simulink model "CMOS_Kernel_Memory_Sync"  (R2023b)
settings: Solver=VariableStepAuto  StartTime=0.0  StopTime=30000000  RelTol=1e-3
values from neighbouring files (symbols this model uses):
  AmountOfPixelsPerScanline = 400    [Kernel_Setup_Script.m]
  AmountOfRamBlocksScanlines = 5    [Kernel_Setup_Script.m]
  AmountOfRamBlocksScanlinesOffset = AmountOfRamBlocksScanlines - 1    (= 4)    [Kernel_Setup_Script.m]
  AmountOfScanlinePixels = 73700    [Kernel_Setup_Script.m]
  AmountOfScanlinePixelsOffset = AmountOfScanlinePixels - 1    (= 73699)    [Kernel_Setup_Script.m]
  AmountOfScanlines = 1100    [Kernel_Setup_Script.m]
  AmountOfScanlinesOffset = AmountOfScanlines - 1    (= 1099)    [Kernel_Setup_Script.m]
  AOPPK_Off = AmountOfPixelsPerScanline - 1    (= 399)    [Kernel_Setup_Script.m]
  AOPPS_Off = AmountOfPixelsPerScanline - 1    (= 399)    [Kernel_Setup_Script.m]
  FramePackOff_0 = FramePackOff_0 - ScanlineFifoCheck    [Kernel_Setup_Script.m]
  FramePackOff_1 = FramePackOff_1 - ScanlineFifoCheck    [Kernel_Setup_Script.m]
  FramePackOff_2 = FramePackOff_2 - ScanlineFifoCheck    [Kernel_Setup_Script.m]
  FramePackOff_3 = FramePackOff_3 - ScanlineFifoCheck    [Kernel_Setup_Script.m]
  FramePackOff_4 = FramePackOff_4 - ScanlineFifoCheck    [Kernel_Setup_Script.m]
  FramePackOff_5 = FramePackOff_5 - ScanlineFifoCheck    [Kernel_Setup_Script.m]
  KernelPackOff_0 = KernelPackOff_0 - KernelBitsPerRow    [Kernel_Setup_Script.m]
  KernelPackOff_1 = KernelPackOff_1 - KernelBitsPerRow    [Kernel_Setup_Script.m]
  KernelPackOff_2 = KernelPackOff_2 - KernelBitsPerRow    [Kernel_Setup_Script.m]
  KernelPackOff_3 = KernelPackOff_3 - KernelBitsPerRow    [Kernel_Setup_Script.m]
  Slice59DownTo48Top = (MsbOffset - (ScanlinePixelBitSizeController*1))    (= 59)    [Kernel_Setup_Script.m]
  Slice71DownTo60Top = (MsbOffset - (ScanlinePixelBitSizeController*0))    (= 71)    [Kernel_Setup_Script.m]
  TotalSectionsForFrames = AmountOfScanlines/AmountOfRamBlocksScanlines    (= 220)    [Kernel_Setup_Script.m]
  UltraRamRows = AmountOfPixelsPerScanline/ScanlineFifoCheck    [Kernel_Setup_Script.m]
  UltraRamRowsCeil = ceil(AmountOfPixelsPerScanline/ScanlineFifoCheck)    [Kernel_Setup_Script.m]
  UltraRamRowsKernel = AmountOfPixelsPerScanline/KernelBitsPerRow    (= 100)    [Kernel_Setup_Script.m]
  UltraRamRowsKernelCeil = ceil(AmountOfPixelsPerScanline/KernelBitsPerRow)    [Kernel_Setup_Script.m]
  UltraRamRowsMemorySectionOffset = UltraRamRowsCeil*AmountOfRamBlocksScanlines    [Kernel_Setup_Script.m]
  UltraRamRowsOffset = UltraRamRowsCeil - 1    [Kernel_Setup_Script.m]
undefined symbols (not defined in the file or in its folder): c, Down, sfvc784, Up, xck26
libraries: hdlBasic x4512, vmcUtilities x1
(part 12 of 39)

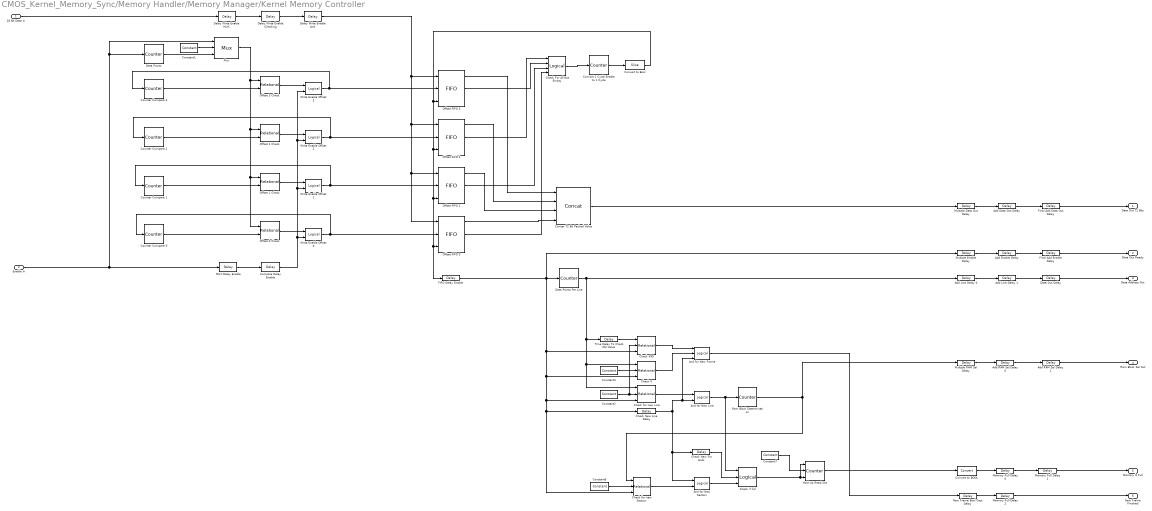
== system CMOS_Kernel_Memory_Sync/Memory Handler/Memory Manager/Kernel Memory Controller ==
  18 Bit Data In : Inport
  Enable In : Inport  Port=2
  Add Data Out Delay : hdlBasic/Delay  rst=off  en=off  latency=1  reg_retiming=off  XmcBlockStatus=1  maskContainerNames=group1  block_type=delay  block_config=sysgen:Delay_config
  Add Enable Delay : hdlBasic/Delay  rst=off  en=off  latency=1  reg_retiming=off  XmcBlockStatus=1  maskContainerNames=group1  block_type=delay  block_config=sysgen:Delay_config
  Add Line Delay 0 : hdlBasic/Delay  rst=off  en=off  latency=3  reg_retiming=off  XmcBlockStatus=1  maskContainerNames=group1  block_type=delay  block_config=sysgen:Delay_config
  Add Line Delay 1 : hdlBasic/Delay  rst=off  en=off  latency=1  reg_retiming=off  XmcBlockStatus=1  maskContainerNames=group1  block_type=delay  block_config=sysgen:Delay_config
  Add RAM Sel Delay 0 : hdlBasic/Delay  rst=off  en=off  latency=1  reg_retiming=off  XmcBlockStatus=1  maskContainerNames=group1  block_type=delay  block_config=sysgen:Delay_config
  Add RAM Sel Delay 1 : hdlBasic/Delay  rst=off  en=off  latency=1  reg_retiming=off  XmcBlockStatus=1  maskContainerNames=group1  block_type=delay  block_config=sysgen:Delay_config
  And for New Frame : hdlBasic/Logical  logical_function=AND  inputs=3  en=off  latency=1  precision=Full  arith_type=Unsigned  n_bits=16  bin_pt=0  align_bp=on  overflow=[]  quantization=[]  XmcBlockStatus=1  maskContainerNames=tabcontainer1  block_type=logical  block_config=sysgen:Logical_config
  And for New Line : hdlBasic/Logical  logical_function=AND  inputs=2  en=off  latency=1  precision=Full  arith_type=Unsigned  n_bits=16  bin_pt=0  align_bp=on  overflow=[]  quantization=[]  XmcBlockStatus=1  maskContainerNames=tabcontainer1  block_type=logical  block_config=sysgen:Logical_config
  And for New Section : hdlBasic/Logical  logical_function=AND  inputs=2  en=off  latency=1  precision=Full  arith_type=Unsigned  n_bits=16  bin_pt=0  align_bp=on  overflow=[]  quantization=[]  XmcBlockStatus=1  maskContainerNames=tabcontainer1  block_type=logical  block_config=sysgen:Logical_config
  Check 0 : hdlBasic/Relational  mode=a=b  op_type=Bool  en=on  latency=1  XmcBlockStatus=1  maskContainerNames=tabcontainer1  block_type=relational  block_config=sysgen:Relational_config
  Check 499 : hdlBasic/Relational  mode=a=b  op_type=Bool  en=on  latency=1  XmcBlockStatus=1  maskContainerNames=tabcontainer1  block_type=relational  block_config=sysgen:Relational_config
  Check For All Not Empty : hdlBasic/Logical  logical_function=NOR  inputs=4  en=off  latency=1  precision=Full  arith_type=Unsigned  n_bits=16  bin_pt=0  align_bp=on  overflow=[]  quantization=[]  XmcBlockStatus=1  maskContainerNames=tabcontainer1  block_type=logical  block_config=sysgen:Logical_config
  Check New For Ands : hdlBasic/Delay  rst=off  en=off  latency=1  reg_retiming=off  XmcBlockStatus=1  maskContainerNames=group1  block_type=delay  block_config=sysgen:Delay_config
  Check New Line Delay : hdlBasic/Delay  rst=off  en=off  latency=1  reg_retiming=off  XmcBlockStatus=1  maskContainerNames=group1  block_type=delay  block_config=sysgen:Delay_config
  Check for new Line : hdlBasic/Relational  mode=a=b  op_type=Bool  en=on  latency=1  XmcBlockStatus=1  maskContainerNames=tabcontainer1  block_type=relational  block_config=sysgen:Relational_config
  Check for new Section : hdlBasic/Relational  mode=a=b  op_type=Bool  en=on  latency=1  XmcBlockStatus=1  maskContainerNames=tabcontainer1  block_type=relational  block_config=sysgen:Relational_config
  Check if full : hdlBasic/Logical  logical_function=AND  inputs=3  en=off  latency=1  precision=Full  arith_type=Unsigned  n_bits=16  bin_pt=0  align_bp=on  overflow=[]  quantization=[]  XmcBlockStatus=1  maskContainerNames=tabcontainer1  block_type=logical  block_config=sysgen:Logical_config
  Compare Delay Enable : hdlBasic/Delay  rst=off  en=off  latency=1  reg_retiming=off  XmcBlockStatus=1  maskContainerNames=group1  block_type=delay  block_config=sysgen:Delay_config
  Concat 72 Bit Packed Value : hdlBasic/Concat  num_inputs=4  XmcBlockStatus=1  maskContainerNames=group1  block_type=concat  block_config=sysgen:Concat_config
  Constant1 : hdlBasic/Constant  const=AOPPK_Off + 1  gui_display_data_type=Fixed-point  arith_type=Unsigned  n_bits=ceil(log2(AmountOfPixelsPerScanline + 1))  bin_pt=0  preci_type=Single  exp_width=8  frac_width=24  explicit_period=off  period=1  XmcBlockStatus=1  maskContainerNames=tabcontainer1  block_type=constant  block_config=sysgen:Constant_config
  Constant2 : hdlBasic/Constant  const=499  gui_display_data_type=Fixed-point  arith_type=Unsigned  n_bits=ceil(log2(UltraRamRowsKernel))+5  bin_pt=0  preci_type=Single  exp_width=8  frac_width=24  explicit_period=off  period=1  XmcBlockStatus=1  maskContainerNames=tabcontainer1  block_type=constant  block_config=sysgen:Constant_config
  Constant3 : hdlBasic/Constant  const=0  gui_display_data_type=Fixed-point  arith_type=Unsigned  n_bits=1  bin_pt=0  preci_type=Single  exp_width=8  frac_width=24  explicit_period=off  period=1  XmcBlockStatus=1  maskContainerNames=tabcontainer1  block_type=constant  block_config=sysgen:Constant_config
  Constant6 : hdlBasic/Constant  const=AmountOfRamBlocksScanlinesOffset  gui_display_data_type=Fixed-point  arith_type=Unsigned  n_bits=ceil(log2(AmountOfRamBlocksScanlines))  bin_pt=0  preci_type=Single  exp_width=8  frac_width=24  explicit_period=off  period=1  XmcBlockStatus=1  maskContainerNames=tabcontainer1  block_type=constant  block_config=sysgen:Constant_config
  Constant7 : hdlBasic/Constant  const=1  gui_display_data_type=Fixed-point  arith_type=Unsigned  n_bits=1  bin_pt=0  preci_type=Single  exp_width=8  frac_width=24  explicit_period=off  period=1  XmcBlockStatus=1  maskContainerNames=tabcontainer1  block_type=constant  block_config=sysgen:Constant_config
  Convert 2 Cycle Enable to 1 Cycle : hdlBasic/Counter  cnt_type=Count limited  cnt_to=2  operation=Up  start_count=0  cnt_by_val=1  arith_type=Unsigned  n_bits=2  bin_pt=0  load_pin=off  rst=off  en=on  explicit_period=Explicit  period=1  use_behavioral_HDL=off  implementation=Fabric  XmcBlockStatus=1  maskContainerNames=group1  block_type=counter  block_config=sysgen:Counter_config  block_width=531  block_height=1023
  Convert to BOOL : hdlBasic/Convert  gui_display_data_type=Boolean  arith_type=Boolean  n_bits=16  bin_pt=14  float_type=Single  exp_bits=8  fraction_bits=24  quantization=Truncate  overflow=Wrap  en=off  latency=3  pipeline=off  XmcBlockStatus=1  maskContainerNames=group2  block_type=convert  block_config=sysgen:Convert_config  block_width=595  block_height=885
  Convert to Bool : hdlBasic/Slice  nbits=1  boolean_output=on  mode=Upper Bit Location + Width  bit1=0  base1=LSB of Input  bit0=0  base0=LSB of Input  XmcBlockStatus=1  maskContainerNames=group1  block_type=slice  block_config=sysgen:Slice_config
  "Counter Compare 0  " : hdlBasic/Counter  cnt_type=Count limited  cnt_to=KernelPackOff_0  operation=Up  start_count=0  cnt_by_val=4  arith_type=Unsigned  n_bits=ceil(log2(KernelPackOff_0+1))  bin_pt=0  load_pin=off  rst=off  en=on  explicit_period=Explicit  period=1  use_behavioral_HDL=off  implementation=Fabric  XmcBlockStatus=1  maskContainerNames=group1  block_type=counter  block_config=sysgen:Counter_config  block_width=531  block_height=1023
  Counter Compare 1 : hdlBasic/Counter  cnt_type=Count limited  cnt_to=KernelPackOff_1  operation=Up  start_count=1  cnt_by_val=4  arith_type=Unsigned  n_bits=ceil(log2(KernelPackOff_1+1))  bin_pt=0  load_pin=off  rst=off  en=on  explicit_period=Explicit  period=1  use_behavioral_HDL=off  implementation=Fabric  XmcBlockStatus=1  maskContainerNames=group1  block_type=counter  block_config=sysgen:Counter_config  block_width=531  block_height=1023
  Counter Compare 2 : hdlBasic/Counter  cnt_type=Count limited  cnt_to=KernelPackOff_2  operation=Up  start_count=2  cnt_by_val=4  arith_type=Unsigned  n_bits=ceil(log2(KernelPackOff_2+1))  bin_pt=0  load_pin=off  rst=off  en=on  explicit_period=Explicit  period=1  use_behavioral_HDL=off  implementation=Fabric  XmcBlockStatus=1  maskContainerNames=group1  block_type=counter  block_config=sysgen:Counter_config  block_width=531  block_height=1023
  Counter Compare 3 : hdlBasic/Counter  cnt_type=Count limited  cnt_to=KernelPackOff_3  operation=Up  start_count=3  cnt_by_val=4  arith_type=Unsigned  n_bits=ceil(log2(KernelPackOff_3+1))  bin_pt=0  load_pin=off  rst=off  en=on  explicit_period=Explicit  period=1  use_behavioral_HDL=off  implementation=Fabric  XmcBlockStatus=1  maskContainerNames=group1  block_type=counter  block_config=sysgen:Counter_config  block_width=531  block_height=1023
  Data Out Delay : hdlBasic/Delay  rst=off  en=off  latency=1  reg_retiming=off  XmcBlockStatus=1  maskContainerNames=group1  block_type=delay  block_config=sysgen:Delay_config
  Data Points : hdlBasic/Counter  cnt_type=Count limited  cnt_to=AOPPK_Off  operation=Up  start_count=0  cnt_by_val=1  arith_type=Unsigned  n_bits=ceil(log2(AmountOfPixelsPerScanline))  bin_pt=0  load_pin=off  rst=off  en=on  explicit_period=Explicit  period=1  use_behavioral_HDL=off  implementation=Fabric  XmcBlockStatus=1  maskContainerNames=group1  block_type=counter  block_config=sysgen:Counter_config  block_width=531  block_height=1023
  Data Points Per Line : hdlBasic/Counter  cnt_type=Count limited  cnt_to=499  operation=Up  start_count=0  cnt_by_val=1  arith_type=Unsigned  n_bits=ceil(log2(UltraRamRowsKernel)) +2  bin_pt=0  load_pin=off  rst=off  en=on  explicit_period=Explicit  period=1  use_behavioral_HDL=off  implementation=Fabric  XmcBlockStatus=1  maskContainerNames=group1  block_type=counter  block_config=sysgen:Counter_config  block_width=531  block_height=1023
  Delay Write Enable And : hdlBasic/Delay  rst=off  en=off  latency=1  reg_retiming=off  XmcBlockStatus=1  maskContainerNames=group1  block_type=delay  block_config=sysgen:Delay_config
  Delay Write Enable Checking : hdlBasic/Delay  rst=off  en=off  latency=1  reg_retiming=off  XmcBlockStatus=1  maskContainerNames=group1  block_type=delay  block_config=sysgen:Delay_config
  Delay Write Enable MUX : hdlBasic/Delay  rst=off  en=off  latency=1  reg_retiming=off  XmcBlockStatus=1  maskContainerNames=group1  block_type=delay  block_config=sysgen:Delay_config
  FIFO Delay Enable : hdlBasic/Delay  rst=off  en=off  latency=1  reg_retiming=off  XmcBlockStatus=1  maskContainerNames=group1  block_type=delay  block_config=sysgen:Delay_config
  Final Add Data Out Delay : hdlBasic/Delay  rst=off  en=off  latency=1  reg_retiming=off  XmcBlockStatus=1  maskContainerNames=group1  block_type=delay  block_config=sysgen:Delay_config
  Final Add Enable Delay : hdlBasic/Delay  rst=off  en=off  latency=1  reg_retiming=off  XmcBlockStatus=1  maskContainerNames=group1  block_type=delay  block_config=sysgen:Delay_config
  Hold Up Read Out : hdlBasic/Counter  cnt_type=Free running  cnt_to=1  operation=Up  start_count=0  cnt_by_val=1  arith_type=Unsigned  n_bits=1  bin_pt=0  load_pin=on  rst=off  en=on  explicit_period=Explicit  period=1  use_behavioral_HDL=off  implementation=Fabric  XmcBlockStatus=1  maskContainerNames=group1  block_type=counter  block_config=sysgen:Counter_config  block_width=531  block_height=1023
  MUX Delay Enable : hdlBasic/Delay  rst=off  en=off  latency=1  reg_retiming=off  XmcBlockStatus=1  maskContainerNames=group1  block_type=delay  block_config=sysgen:Delay_config
  Memory Full Delay 0 : hdlBasic/Delay  rst=off  en=off  latency=1  reg_retiming=off  XmcBlockStatus=1  maskContainerNames=group1  block_type=delay  block_config=sysgen:Delay_config
  Memory Full Delay 1 : hdlBasic/Delay  rst=off  en=off  latency=1  reg_retiming=off  XmcBlockStatus=1  maskContainerNames=group1  block_type=delay  block_config=sysgen:Delay_config
  Memory Full Delay 2 : hdlBasic/Delay  rst=off  en=off  latency=1  reg_retiming=off  XmcBlockStatus=1  maskContainerNames=group1  block_type=delay  block_config=sysgen:Delay_config
  Multiple Data Out Delay : hdlBasic/Delay  rst=off  en=off  latency=3  reg_retiming=off  XmcBlockStatus=1  maskContainerNames=group1  block_type=delay  block_config=sysgen:Delay_config
  Multiple Enable Delay : hdlBasic/Delay  rst=off  en=off  latency=3  reg_retiming=off  XmcBlockStatus=1  maskContainerNames=group1  block_type=delay  block_config=sysgen:Delay_config
  Multiple RAM Sel Delay : hdlBasic/Delay  rst=off  en=off  latency=3  reg_retiming=off  XmcBlockStatus=1  maskContainerNames=group1  block_type=delay  block_config=sysgen:Delay_config
  Mux : hdlBasic/Mux  inputs=2  en=off  latency=1  precision=Full  arith_type=Unsigned  n_bits=16  bin_pt=14  quantization=Truncate  overflow=Wrap  XmcBlockStatus=1  maskContainerNames=tabcontainer1  block_type=mux  block_config=sysgen:Mux_config
  New Frame Bool Cast Delay : hdlBasic/Delay  rst=off  en=off  latency=3  reg_retiming=off  XmcBlockStatus=1  maskContainerNames=group1  block_type=delay  block_config=sysgen:Delay_config
  Offset 0 Check : hdlBasic/Relational  mode=a=b  op_type=Bool  en=off  latency=1  XmcBlockStatus=1  maskContainerNames=tabcontainer1  block_type=relational  block_config=sysgen:Relational_config
  Offset 1 Check : hdlBasic/Relational  mode=a=b  op_type=Bool  en=off  latency=1  XmcBlockStatus=1  maskContainerNames=tabcontainer1  block_type=relational  block_config=sysgen:Relational_config
  Offset 2 Check : hdlBasic/Relational  mode=a=b  op_type=Bool  en=off  latency=1  XmcBlockStatus=1  maskContainerNames=tabcontainer1  block_type=relational  block_config=sysgen:Relational_config
  Offset 3 Check : hdlBasic/Relational  mode=a=b  op_type=Bool  en=off  latency=1  XmcBlockStatus=1  maskContainerNames=tabcontainer1  block_type=relational  block_config=sysgen:Relational_config
  Offset FIFO {0..3} (4 alike) : hdlBasic/FIFO  mem_type=Block RAM  performance_options=Standard_FIFO  embedded_registers=off  depth=16  use_asym_data_widths=off  asym_read_width=32  percent_nbits=4  rst=off  rst_latency=2  en=off  use_dcount=off  use_percent_full_port=off  use_almost_empty=off  almost_empty_thresh=2  use_almost_full=off  use_rd_rst_busy=off  use_wr_rst_busy=off  almost_full_thresh=14  almost_empty_offset=[]  almost_full_offset=[]  explicit_period=off  period=[]  store_only_valid=[]  init_zero=[]  simulation_type=fast_sim  XmcBlockStatus=1  maskContainerNames=tabcontainer1  block_type=fifo  block_config=sysgen:FIFO_config  block_width=538  block_height=997
      settings: infoedit=[]
  Ram Block Determination : hdlBasic/Counter  cnt_type=Count limited  cnt_to=AmountOfRamBlocksScanlinesOffset  operation=Up  start_count=0  cnt_by_val=1  arith_type=Unsigned  n_bits=ceil(log2(AmountOfRamBlocksScanlines))  bin_pt=0  load_pin=off  rst=off  en=on  explicit_period=Explicit  period=1  use_behavioral_HDL=off  implementation=Fabric  XmcBlockStatus=1  maskContainerNames=group1  block_type=counter  block_config=sysgen:Counter_config  block_width=531  block_height=1023
  Time Delay To Check Old Value : hdlBasic/Delay  rst=off  en=off  latency=3  reg_retiming=off  XmcBlockStatus=1  maskContainerNames=group1  block_type=delay  block_config=sysgen:Delay_config
  Write Enable Offset {0..3} (4 alike) : hdlBasic/Logical  logical_function=AND  inputs=2  en=off  latency=1  precision=Full  arith_type=Unsigned  n_bits=16  bin_pt=0  align_bp=on  overflow=[]  quantization=[]  XmcBlockStatus=1  maskContainerNames=tabcontainer1  block_type=logical  block_config=sysgen:Logical_config
  Data Out 72 Bits : Outport
  Data Out Ready : Outport  Port=2
  Data Address Out : Outport  Port=3
  Ram Block Sel Out : Outport  Port=4
  Memory Is Full : Outport  Port=5
  New Frame Finished : Outport  Port=6
  wires:
  FIFO Delay Enable/1 -> Multiple Enable Delay/1, Check 499/3, Check 0/3, Check for new Line/3, Check New Line Delay/1, Check for new Section/3, Data Points Per Line/1
  Add RAM Sel Delay 1/1 -> Ram Block Sel Out/1
  Add Line Delay 0/1 -> Add Line Delay 1/1
  Offset FIFO 3/2 -> Check For All Not Empty/2
  Convert to Bool/1 -> FIFO Delay Enable/1, Offset FIFO 0/3, Offset FIFO 1/3, Offset FIFO 2/3, Offset FIFO 3/3
  Add RAM Sel Delay 0/1 -> Add RAM Sel Delay 1/1
  Check New Line Delay/1 -> And for New Section/1, Check New For Ands/1, And for New Line/2, And for New Frame/3
  Constant2/1 -> Check for new Line/2, Check 499/2
  Offset FIFO 0/2 -> Check For All Not Empty/4
  Constant6/1 -> Check for new Section/2
  Add Enable Delay/1 -> Final Add Enable Delay/1
  Data Points Per Line/1 -> Check 0/1, Check for new Line/1, Time Delay To Check Old Value/1, Add Line Delay 0/1
  Check For All Not Empty/1 -> Convert 2 Cycle Enable to 1 Cycle/1
  Add Data Out Delay/1 -> Final Add Data Out Delay/1
  Multiple RAM Sel Delay/1 -> Add RAM Sel Delay 0/1
  Offset FIFO 2/2 -> Check For All Not Empty/1
  Multiple Enable Delay/1 -> Add Enable Delay/1
  Offset 0 Check/1 -> Write Enable Offset 0/1
  Offset FIFO 1/2 -> Check For All Not Empty/3
  Offset 1 Check/1 -> Write Enable Offset 1/1
  And for New Line/1 -> Check if full/1, Ram Block Determination/1
  Convert 2 Cycle Enable to 1 Cycle/1 -> Convert to Bool/1
  Offset 2 Check/1 -> Write Enable Offset 2/1
  Concat 72 Bit Packed Value/1 -> Multiple Data Out Delay/1
  Ram Block Determination/1 -> Check for new Section/1, Multiple RAM Sel Delay/1
  Counter Compare 2/1 -> Offset 2 Check/2
  Counter Compare 1/1 -> Offset 1 Check/2
  "Counter Compare 0  "/1 -> Offset 0 Check/2
  Add Line Delay 1/1 -> Data Out Delay/1
  Multiple Data Out Delay/1 -> Add Data Out Delay/1
  Final Add Data Out Delay/1 -> Data Out 72 Bits/1
  Final Add Enable Delay/1 -> Data Out Ready/1
  Data Out Delay/1 -> Data Address Out/1
  Memory Full Delay 1/1 -> Memory Is Full/1
  Check if full/1 -> Hold Up Read Out/1, Hold Up Read Out/3
  Hold Up Read Out/1 -> Convert to BOOL/1
  Convert to BOOL/1 -> Memory Full Delay 0/1
  Constant7/1 -> Hold Up Read Out/2
  Memory Full Delay 0/1 -> Memory Full Delay 1/1
  Offset FIFO 0/1 -> Concat 72 Bit Packed Value/4
  Offset FIFO 1/1 -> Concat 72 Bit Packed Value/3
  Offset FIFO 2/1 -> Concat 72 Bit Packed Value/2
  Offset FIFO 3/1 -> Concat 72 Bit Packed Value/1
  Offset 3 Check/1 -> Write Enable Offset 3/1
  Counter Compare 3/1 -> Offset 3 Check/2
  Check for new Section/1 -> And for New Section/2
  And for New Section/1 -> Check if full/3
  Check New For Ands/1 -> Check if full/2
  Check for new Line/1 -> And for New Line/1
  Memory Full Delay 2/1 -> New Frame Finished/1
  Time Delay To Check Old Value/1 -> Check 499/1
  Check 499/1 -> And for New Frame/1
  Check 0/1 -> And for New Frame/2
  Constant3/1 -> Check 0/2
  And for New Frame/1 -> New Frame Bool Cast Delay/1
  New Frame Bool Cast Delay/1 -> Memory Full Delay 2/1
  Write Enable Offset 0/1 -> "Counter Compare 0  "/1, Offset FIFO 0/2
  Write Enable Offset 1/1 -> Counter Compare 1/1, Offset FIFO 1/2
  Write Enable Offset 3/1 -> Counter Compare 3/1, Offset FIFO 3/2
  Write Enable Offset 2/1 -> Counter Compare 2/1, Offset FIFO 2/2
  Delay Write Enable And/1 -> Offset FIFO 0/1, Offset FIFO 1/1, Offset FIFO 2/1, Offset FIFO 3/1
  Compare Delay Enable/1 -> Write Enable Offset 0/2, Write Enable Offset 1/2, Write Enable Offset 2/2, Write Enable Offset 3/2
  Delay Write Enable Checking/1 -> Delay Write Enable And/1
  Constant1/1 -> Mux/2
  Data Points/1 -> Mux/3
  Mux/1 -> Offset 3 Check/1, Offset 2 Check/1, Offset 0 Check/1, Offset 1 Check/1
  Delay Write Enable MUX/1 -> Delay Write Enable Checking/1
  MUX Delay Enable/1 -> Compare Delay Enable/1
  18 Bit Data In/1 -> Delay Write Enable MUX/1
  Enable In/1 -> Mux/1, Data Points/1, MUX Delay Enable/1

== system CMOS_Kernel_Memory_Sync/Memory Handler/Memory Manager/Kernel Memory Subsystem ==
  Read Address : Inport
  Read Enable : Inport  Port=2
  Write Address : Inport  Port=3
  Write Data to RAM Sel : Inport  Port=4
  Data To Write : Inport  Port=5
  Write Enable : Inport  Port=6
  Convert to BOOL : hdlBasic/Convert  gui_display_data_type=Boolean  arith_type=Boolean  n_bits=16  bin_pt=14  float_type=Single  exp_bits=8  fraction_bits=24  quantization=Truncate  overflow=Wrap  en=off  latency=1  pipeline=off  XmcBlockStatus=1  maskContainerNames=group2  block_type=convert  block_config=sysgen:Convert_config  block_width=595  block_height=885
  Dual Port RAM {0..4} (5 alike) : hdlBasic/Dual Port RAM  depth=KernelRamDepth  initVector=sin(pi*(0:15)/16)  distributed_mem=Ultra RAM  init_a=0  init_b=0  rst_a=off  rst_b=off  en_a=on  en_b=on  latency=1  write_mode_A=Read After Write  write_mode_B=Read After Write  explicit_period=[]  period=[]  simulation_type=fast_sim  XmcBlockStatus=1  maskContainerNames=tabcontainer1  block_type=dpram  block_config=sysgen:Dpram_config  optimize=Area
      settings: infoedit=[]
  RAM Selector 0 : Subsystem
      settings: RTWMemSecFuncInitTerm=Inherit fRAM model  RTWMemSecFuncExecute=Inherit fRAM model  RTWMemSecDataConstants=Inherit fRAM model  RTWMemSecDataInternal=Inherit fRAM model  RTWMemSecDataParameters=Inherit fRAM model
  RAM Selector 1 : Subsystem
      settings: RTWMemSecFuncInitTerm=Inherit fRAM model  RTWMemSecFuncExecute=Inherit fRAM model  RTWMemSecDataConstants=Inherit fRAM model  RTWMemSecDataInternal=Inherit fRAM model  RTWMemSecDataParameters=Inherit fRAM model
  RAM Selector 2 : Subsystem
      settings: RTWMemSecFuncInitTerm=Inherit fRAM model  RTWMemSecFuncExecute=Inherit fRAM model  RTWMemSecDataConstants=Inherit fRAM model  RTWMemSecDataInternal=Inherit fRAM model  RTWMemSecDataParameters=Inherit fRAM model
  Read Constant : hdlBasic/Constant  const=0  gui_display_data_type=Boolean  arith_type=Boolean  n_bits=16  bin_pt=14  preci_type=Single  exp_width=8  frac_width=24  explicit_period=off  period=1  XmcBlockStatus=1  maskContainerNames=tabcontainer1  block_type=constant  block_config=sysgen:Constant_config
  Write Constant : hdlBasic/Constant  const=1.0  gui_display_data_type=Boolean  arith_type=Boolean  n_bits=16  bin_pt=14  preci_type=Single  exp_width=8  frac_width=24  explicit_period=off  period=1  XmcBlockStatus=1  maskContainerNames=tabcontainer1  block_type=constant  block_config=sysgen:Constant_config
  RAM 0 Out : Outport
  RAM 1 Out : Outport  Port=2
  RAM 2 Out : Outport  Port=3
  RAM 3 Out : Outport  Port=4
  RAM 4 Out : Outport  Port=5
  Valid : Outport  Port=6
  wires:
  RAM Selector 2/1(Out RAM 0) -> Dual Port RAM 0/8
  Dual Port RAM 1/1 -> RAM 1 Out/1
  RAM Selector 0/5(Out RAM 4) -> Dual Port RAM 4/4
  Write Constant/1 -> Dual Port RAM 4/6, Dual Port RAM 3/6, Dual Port RAM 2/6, Dual Port RAM 1/6, Dual Port RAM 0/6
  Read Constant/1 -> Dual Port RAM 4/3, Dual Port RAM 3/3, Dual Port RAM 2/3, Dual Port RAM 1/3, Dual Port RAM 0/3
  RAM Selector 1/4(Out RAM 3) -> Dual Port RAM 3/2, Dual Port RAM 3/5
  RAM Selector 0/2(Out RAM 1) -> Dual Port RAM 1/4
  RAM Selector 2/5(Out RAM 4) -> Dual Port RAM 4/8
  RAM Selector 0/4(Out RAM 3) -> Dual Port RAM 3/4
  RAM Selector 1/1(Out RAM 0) -> Dual Port RAM 0/2, Dual Port RAM 0/5
  RAM Selector 1/2(Out RAM 1) -> Dual Port RAM 1/2, Dual Port RAM 1/5
  RAM Selector 1/5(Out RAM 4) -> Dual Port RAM 4/2, Dual Port RAM 4/5
  RAM Selector 1/3(Out RAM 2) -> Dual Port RAM 2/2, Dual Port RAM 2/5
  Dual Port RAM 4/1 -> RAM 4 Out/1
  RAM Selector 0/1(Out RAM 0) -> Dual Port RAM 0/4
  RAM Selector 0/3(Out RAM 2) -> Dual Port RAM 2/4
  RAM Selector 2/2(Out RAM 1) -> Dual Port RAM 1/8
  RAM Selector 2/4(Out RAM 3) -> Dual Port RAM 3/8
  RAM Selector 2/3(Out RAM 2) -> Dual Port RAM 2/8
  Dual Port RAM 3/1 -> RAM 3 Out/1
  Dual Port RAM 2/1 -> RAM 2 Out/1
  Dual Port RAM 0/1 -> RAM 0 Out/1
  Write Enable/1 -> RAM Selector 2/1(Data In)
  Data To Write/1 -> RAM Selector 1/1(Data In)
  Write Address/1 -> RAM Selector 0/1(Data In)
  Write Data to RAM Sel/1 -> RAM Selector 0/2(RAM Select), RAM Selector 2/2(RAM Select), RAM Selector 1/2(RAM Select)
  Read Address/1 -> Dual Port RAM 0/1, Dual Port RAM 4/1, Dual Port RAM 3/1, Dual Port RAM 2/1, Dual Port RAM 1/1
  Read Enable/1 -> Convert to BOOL/1, Dual Port RAM 4/7, Dual Port RAM 3/7, Dual Port RAM 2/7, Dual Port RAM 1/7, Dual Port RAM 0/7
  Convert to BOOL/1 -> Valid/1

== system CMOS_Kernel_Memory_Sync/Memory Handler/Memory Manager/Memory Sync ==
  Frame Memory Full : Inport
  Kernel Memory Full : Inport  Port=2
  New Frame : Inport  Port=3
  Reset : Inport  Port=4
  Add Frame Memory Address Delay : hdlBasic/Delay  rst=off  en=off  latency=1  reg_retiming=off  XmcBlockStatus=1  maskContainerNames=group1  block_type=delay  block_config=sysgen:Delay_config
  Add Frame Read Enable Delay : hdlBasic/Delay  rst=off  en=off  latency=1  reg_retiming=off  XmcBlockStatus=1  maskContainerNames=group1  block_type=delay  block_config=sysgen:Delay_config
  Add Kernel Read Enable Delay : hdlBasic/Delay  rst=off  en=off  latency=1  reg_retiming=off  XmcBlockStatus=1  maskContainerNames=group1  block_type=delay  block_config=sysgen:Delay_config
  Add Offset : hdlBasic/AddSub  mode=Addition  use_carryin=off  use_carryout=off  en=off  latency=1  precision=Full  arith_type=Unsigned  n_bits=16  bin_pt=14  quantization=Truncate  overflow=Wrap  use_behavioral_HDL=off  hw_selection=Fabric  pipelined=off  XmcBlockStatus=1  maskContainerNames=tabcontainer1  block_type=addsub  block_config=sysgen:Addsub_config
  Check If at Reset Point : hdlBasic/Relational  mode=a=b  op_type=Bool  en=off  latency=1  XmcBlockStatus=1  maskContainerNames=tabcontainer1  block_type=relational  block_config=sysgen:Relational_config
  Check Last Address1 : hdlBasic/Relational  mode=a=b  op_type=Bool  en=off  latency=1  XmcBlockStatus=1  maskContainerNames=tabcontainer1  block_type=relational  block_config=sysgen:Relational_config
  Check Once1 : hdlBasic/Logical  logical_function=AND  inputs=2  en=off  latency=1  precision=Full  arith_type=Unsigned  n_bits=16  bin_pt=0  align_bp=on  overflow=[]  quantization=[]  XmcBlockStatus=1  maskContainerNames=tabcontainer1  block_type=logical  block_config=sysgen:Logical_config
  Check if 2 Frame Sync : hdlBasic/Relational  mode=a!=b  op_type=Bool  en=off  latency=1  XmcBlockStatus=1  maskContainerNames=tabcontainer1  block_type=relational  block_config=sysgen:Relational_config
  Check to Remove Offset : hdlBasic/Relational  mode=a>b  op_type=Bool  en=off  latency=1  XmcBlockStatus=1  maskContainerNames=tabcontainer1  block_type=relational  block_config=sysgen:Relational_config
  Constant1 : hdlBasic/Constant  const=2  gui_display_data_type=Fixed-point  arith_type=Unsigned  n_bits=2  bin_pt=0  preci_type=Single  exp_width=8  frac_width=24  explicit_period=off  period=1  XmcBlockStatus=1  maskContainerNames=tabcontainer1  block_type=constant  block_config=sysgen:Constant_config
  Constant2 : hdlBasic/Constant  const=AmountOfScanlinePixelsOffset - 3  gui_display_data_type=Fixed-point  arith_type=Unsigned  n_bits=ceil(log2(AmountOfScanlinePixels))  bin_pt=0  preci_type=Single  exp_width=8  frac_width=24  explicit_period=off  period=1  XmcBlockStatus=1  maskContainerNames=tabcontainer1  block_type=constant  block_config=sysgen:Constant_config
  Constant3 : hdlBasic/Constant  const=499  gui_display_data_type=Fixed-point  arith_type=Unsigned  n_bits=ceil(log2(499))  bin_pt=0  preci_type=Single  exp_width=8  frac_width=24  explicit_period=off  period=1  XmcBlockStatus=1  maskContainerNames=tabcontainer1  block_type=constant  block_config=sysgen:Constant_config
  Constant4 : hdlBasic/Constant  const=500  gui_display_data_type=Fixed-point  arith_type=Unsigned  n_bits=ceil(log2(499))  bin_pt=0  preci_type=Single  exp_width=8  frac_width=24  explicit_period=off  period=1  XmcBlockStatus=1  maskContainerNames=tabcontainer1  block_type=constant  block_config=sysgen:Constant_config
  Constant5 : hdlBasic/Constant  const=98  gui_display_data_type=Fixed-point  arith_type=Unsigned  n_bits=8  bin_pt=0  preci_type=Single  exp_width=8  frac_width=24  explicit_period=off  period=1  XmcBlockStatus=1  maskContainerNames=tabcontainer1  block_type=constant  block_config=sysgen:Constant_config
  Count Positive : hdlBasic/Logical  logical_function=OR  inputs=2  en=off  latency=1  precision=Full  arith_type=Unsigned  n_bits=16  bin_pt=0  align_bp=on  overflow=[]  quantization=[]  XmcBlockStatus=1  maskContainerNames=tabcontainer1  block_type=logical  block_config=sysgen:Logical_config
  Count to 3 : hdlBasic/Counter  cnt_type=Count limited  cnt_to=2  operation=Up  start_count=0  cnt_by_val=1  arith_type=Unsigned  n_bits=2  bin_pt=0  load_pin=off  rst=on  en=on  explicit_period=Explicit  period=1  use_behavioral_HDL=off  implementation=Fabric  XmcBlockStatus=1  maskContainerNames=group1  block_type=counter  block_config=sysgen:Counter_config  block_width=531  block_height=1023
  Count to Max Frame Memory : hdlBasic/Counter  cnt_type=Count limited  cnt_to=AmountOfScanlinePixelsOffset  operation=Up  start_count=0  cnt_by_val=1  arith_type=Unsigned  n_bits=ceil(log2(AmountOfScanlinePixels))  bin_pt=0  load_pin=off  rst=off  en=on  explicit_period=Explicit  period=1  use_behavioral_HDL=off  implementation=Fabric  XmcBlockStatus=1  maskContainerNames=group1  block_type=counter  block_config=sysgen:Counter_config  block_width=531  block_height=1023
  Delay1 : hdlBasic/Delay  rst=off  en=off  latency=1  reg_retiming=off  XmcBlockStatus=1  maskContainerNames=group1  block_type=delay  block_config=sysgen:Delay_config
  Enable Circular Buffer State Update : hdlBasic/Delay  rst=off  en=off  latency=4  reg_retiming=off  XmcBlockStatus=1  maskContainerNames=group1  block_type=delay  block_config=sysgen:Delay_config
  Enable Frame Counter : hdlBasic/Logical  logical_function=OR  inputs=3  en=off  latency=1  precision=Full  arith_type=Unsigned  n_bits=16  bin_pt=0  align_bp=on  overflow=[]  quantization=[]  XmcBlockStatus=1  maskContainerNames=tabcontainer1  block_type=logical  block_config=sysgen:Logical_config
  Frame Counter All On : hdlBasic/Logical  logical_function=AND  inputs=2  en=off  latency=1  precision=Full  arith_type=Unsigned  n_bits=16  bin_pt=0  align_bp=on  overflow=[]  quantization=[]  XmcBlockStatus=1  maskContainerNames=tabcontainer1  block_type=logical  block_config=sysgen:Logical_config
  Hold Up Read Out Frame : hdlBasic/Counter  cnt_type=Count limited  cnt_to=1  operation=Up/Down  start_count=0  cnt_by_val=1  arith_type=Unsigned  n_bits=1  bin_pt=0  load_pin=off  rst=off  en=on  explicit_period=Explicit  period=1  use_behavioral_HDL=off  implementation=Fabric  XmcBlockStatus=1  maskContainerNames=group1  block_type=counter  block_config=sysgen:Counter_config  block_width=531  block_height=1023
  Kernel Count : hdlBasic/Counter  cnt_type=Count limited  cnt_to=99  operation=Up  start_count=0  cnt_by_val=1  arith_type=Unsigned  n_bits=7  bin_pt=0  load_pin=off  rst=off  en=on  explicit_period=Explicit  period=1  use_behavioral_HDL=off  implementation=Fabric  XmcBlockStatus=1  maskContainerNames=group1  block_type=counter  block_config=sysgen:Counter_config  block_width=531  block_height=1023
  Kernel Count Full : hdlBasic/Counter  cnt_type=Count limited  cnt_to=499  operation=Up  start_count=0  cnt_by_val=1  arith_type=Unsigned  n_bits=9  bin_pt=0  load_pin=off  rst=off  en=on  explicit_period=Explicit  period=1  use_behavioral_HDL=off  implementation=Fabric  XmcBlockStatus=1  maskContainerNames=group1  block_type=counter  block_config=sysgen:Counter_config  block_width=531  block_height=1023
  Kernel Offset : hdlBasic/Counter  cnt_type=Count limited  cnt_to=100  operation=Down  start_count=500  cnt_by_val=100  arith_type=Unsigned  n_bits=9  bin_pt=0  load_pin=off  rst=off  en=on  explicit_period=Explicit  period=1  use_behavioral_HDL=off  implementation=Fabric  XmcBlockStatus=1  maskContainerNames=group1  block_type=counter  block_config=sysgen:Counter_config  block_width=531  block_height=1023
  Logical : hdlBasic/Logical  logical_function=AND  inputs=3  en=off  latency=1  precision=Full  arith_type=Unsigned  n_bits=16  bin_pt=0  align_bp=on  overflow=[]  quantization=[]  XmcBlockStatus=1  maskContainerNames=tabcontainer1  block_type=logical  block_config=sysgen:Logical_config
  Remove Offset Frame Memory Address Delay : hdlBasic/Delay  rst=off  en=off  latency=1  reg_retiming=off  XmcBlockStatus=1  maskContainerNames=group1  block_type=delay  block_config=sysgen:Delay_config
  Remove Offset Frame Memory Address Delay1 : hdlBasic/Delay  rst=off  en=off  latency=1  reg_retiming=off  XmcBlockStatus=1  maskContainerNames=group1  block_type=delay  block_config=sysgen:Delay_config
  Remove Offset Frame Read Enable Delay : hdlBasic/Delay  rst=off  en=off  latency=1  reg_retiming=off  XmcBlockStatus=1  maskContainerNames=group1  block_type=delay  block_config=sysgen:Delay_config
  Remove Offset Frame Read Enable Delay1 : hdlBasic/Delay  rst=off  en=off  latency=1  reg_retiming=off  XmcBlockStatus=1  maskContainerNames=group1  block_type=delay  block_config=sysgen:Delay_config
  Remove Offset Kernel Read Delay : hdlBasic/Delay  rst=off  en=off  latency=1  reg_retiming=off  XmcBlockStatus=1  maskContainerNames=group1  block_type=delay  block_config=sysgen:Delay_config
  Remove Offset MUX : hdlBasic/Mux  inputs=2  en=off  latency=1  precision=Full  arith_type=Unsigned  n_bits=16  bin_pt=14  quantization=Truncate  overflow=Wrap  XmcBlockStatus=1  maskContainerNames=tabcontainer1  block_type=mux  block_config=sysgen:Mux_config
  Remove Offset MUX Read Delay : hdlBasic/Delay  rst=off  en=off  latency=1  reg_retiming=off  XmcBlockStatus=1  maskContainerNames=group1  block_type=delay  block_config=sysgen:Delay_config
  Remove Offset Original Delay and Cast : hdlBasic/Convert  gui_display_data_type=Fixed-point  arith_type=Unsigned  n_bits=9  bin_pt=0  float_type=Single  exp_bits=8  fraction_bits=24  quantization=Truncate  overflow=Wrap  en=off  latency=1  pipeline=off  XmcBlockStatus=1  maskContainerNames=group2  block_type=convert  block_config=sysgen:Convert_config  block_width=595  block_height=885
  Remove Offset Subtracked Delay and Cast : hdlBasic/Convert  gui_display_data_type=Fixed-point  arith_type=Unsigned  n_bits=9  bin_pt=0  float_type=Single  exp_bits=8  fraction_bits=24  quantization=Truncate  overflow=Wrap  en=off  latency=1  pipeline=off  XmcBlockStatus=1  maskContainerNames=group2  block_type=convert  block_config=sysgen:Convert_config  block_width=595  block_height=885
  Subtrack Delay : hdlBasic/Delay  rst=off  en=off  latency=1  reg_retiming=off  XmcBlockStatus=1  maskContainerNames=group1  block_type=delay  block_config=sysgen:Delay_config
  Subtrack Frame Memory Address Delay : hdlBasic/Delay  rst=off  en=off  latency=1  reg_retiming=off  XmcBlockStatus=1  maskContainerNames=group1  block_type=delay  block_config=sysgen:Delay_config
  Subtrack Frame Read Enable Delay : hdlBasic/Delay  rst=off  en=off  latency=1  reg_retiming=off  XmcBlockStatus=1  maskContainerNames=group1  block_type=delay  block_config=sysgen:Delay_config
  Subtrack Kernel Read Enable Delay : hdlBasic/Delay  rst=off  en=off  latency=1  reg_retiming=off  XmcBlockStatus=1  maskContainerNames=group1  block_type=delay  block_config=sysgen:Delay_config
  Subtrack Offset : hdlBasic/AddSub  mode=Subtraction  use_carryin=off  use_carryout=off  en=off  latency=1  precision=Full  arith_type=Unsigned  n_bits=16  bin_pt=14  quantization=Truncate  overflow=Wrap  use_behavioral_HDL=off  hw_selection=Fabric  pipelined=off  XmcBlockStatus=1  maskContainerNames=tabcontainer1  block_type=addsub  block_config=sysgen:Addsub_config
  Turn On Generator : hdlBasic/Convert  gui_display_data_type=Boolean  arith_type=Boolean  n_bits=16  bin_pt=14  float_type=Single  exp_bits=8  fraction_bits=24  quantization=Truncate  overflow=Wrap  en=off  latency=1  pipeline=off  XmcBlockStatus=1  maskContainerNames=group2  block_type=convert  block_config=sysgen:Convert_config  block_width=595  block_height=885
  Frame Memory Address : Outport
  Frame Read Enable : Outport  Port=2
  Kernel Memory Address : Outport  Port=3
  Kernel Read Enable : Outport  Port=4
  wires:
  Frame Memory Full/1 -> Logical/1
  Kernel Memory Full/1 -> Logical/2
  New Frame/1 -> Logical/3
  Logical/1 -> Count Positive/1, Enable Frame Counter/1
  Count Positive/1 -> Hold Up Read Out Frame/1
  Enable Frame Counter/1 -> Hold Up Read Out Frame/2
  Reset/1 -> Count Positive/2, Enable Frame Counter/2
  Hold Up Read Out Frame/1 -> Turn On Generator/1
  Count to 3/1 -> Check if 2 Frame Sync/2
  Count to Max Frame Memory/1 -> Check Last Address1/1, Add Frame Memory Address Delay/1
  Constant1/1 -> Check if 2 Frame Sync/1
  Check if 2 Frame Sync/1 -> Frame Counter All On/1
  Check Last Address1/1 -> Check Once1/2
  Constant2/1 -> Check Last Address1/2
  Delay1/1 -> Check Once1/1
  Frame Counter All On/1 -> Count to Max Frame Memory/1, Add Frame Read Enable Delay/1, Delay1/1
  Check Once1/1 -> Enable Frame Counter/3, Enable Circular Buffer State Update/1
  Constant5/1 -> Check If at Reset Point/1
  Check If at Reset Point/1 -> Count to 3/1
  Kernel Count/1 -> Check If at Reset Point/2
  Turn On Generator/1 -> Add Kernel Read Enable Delay/1, Kernel Count Full/1, Frame Counter All On/2, Count to 3/2, Kernel Count/1
  Enable Circular Buffer State Update/1 -> Kernel Offset/1
  Kernel Count Full/1 -> Add Offset/1
  Kernel Offset/1 -> Add Offset/2
  Add Kernel Read Enable Delay/1 -> Subtrack Kernel Read Enable Delay/1
  Add Frame Read Enable Delay/1 -> Subtrack Frame Read Enable Delay/1
  Add Frame Memory Address Delay/1 -> Subtrack Frame Memory Address Delay/1
  Add Offset/1 -> Subtrack Offset/1, Subtrack Delay/1
  Subtrack Delay/1 -> Remove Offset Subtracked Delay and Cast/1, Check to Remove Offset/1
  Subtrack Kernel Read Enable Delay/1 -> Remove Offset Kernel Read Delay/1
  Subtrack Frame Read Enable Delay/1 -> Remove Offset Frame Read Enable Delay/1
  Subtrack Frame Memory Address Delay/1 -> Remove Offset Frame Memory Address Delay/1
  Constant3/1 -> Check to Remove Offset/2
  Check to Remove Offset/1 -> Remove Offset MUX/1
  Subtrack Offset/1 -> Remove Offset Original Delay and Cast/1
  Remove Offset Kernel Read Delay/1 -> Remove Offset MUX Read Delay/1
  Remove Offset Original Delay and Cast/1 -> Remove Offset MUX/3
  Remove Offset Subtracked Delay and Cast/1 -> Remove Offset MUX/2
  Remove Offset MUX/1 -> Kernel Memory Address/1
  Remove Offset MUX Read Delay/1 -> Kernel Read Enable/1
  Remove Offset Frame Read Enable Delay/1 -> Remove Offset Frame Read Enable Delay1/1
  Remove Offset Frame Memory Address Delay/1 -> Remove Offset Frame Memory Address Delay1/1
  Constant4/1 -> Subtrack Offset/2
  Remove Offset Frame Memory Address Delay1/1 -> Frame Memory Address/1
  Remove Offset Frame Read Enable Delay1/1 -> Frame Read Enable/1

== system CMOS_Kernel_Memory_Sync/Memory Handler/Memory Manager/Memory Sync Delay Frame Write ==
  Data Out 72 Bits : Inport
  Data Out Ready : Inport  Port=2
  Data Address Out : Inport  Port=3
  Ram Bloack Sel Out : Inport  Port=4
  Delay {0..3} (4 alike) : hdlBasic/Delay  rst=off  en=off  latency=600  reg_retiming=off  XmcBlockStatus=1  maskContainerNames=group1  block_type=delay  block_config=sysgen:Delay_config
  Data To Write : Outport
  Write Enable : Outport  Port=2
  Write Address : Outport  Port=3
  Write Data to RAM Sel : Outport  Port=4
  wires:
  Ram Bloack Sel Out/1 -> Delay 3/1
  Data Address Out/1 -> Delay 2/1
  Delay 0/1 -> Data To Write/1
  Delay 2/1 -> Write Address/1
  Data Out 72 Bits/1 -> Delay 0/1
  Data Out Ready/1 -> Delay 1/1
  Delay 1/1 -> Write Enable/1
  Delay 3/1 -> Write Data to RAM Sel/1

== system CMOS_Kernel_Memory_Sync/Memory Handler/Memory Manager/Memory Sync Delay Frame Write1 ==
  Data Out 72 Bits : Inport
  Data Out Ready : Inport  Port=2
  Data Address Out : Inport  Port=3
  Ram Bloack Sel Out : Inport  Port=4
  Delay {0..3} (4 alike) : hdlBasic/Delay  rst=off  en=off  latency=400  reg_retiming=off  XmcBlockStatus=1  maskContainerNames=group1  block_type=delay  block_config=sysgen:Delay_config
  Data To Write : Outport
  Write Enable : Outport  Port=2
  Write Address : Outport  Port=3
  Write Data to RAM Sel : Outport  Port=4
  wires:
  Ram Bloack Sel Out/1 -> Delay 3/1
  Data Address Out/1 -> Delay 2/1
  Delay 0/1 -> Data To Write/1
  Delay 2/1 -> Write Address/1
  Data Out 72 Bits/1 -> Delay 0/1
  Data Out Ready/1 -> Delay 1/1
  Delay 1/1 -> Write Enable/1
  Delay 3/1 -> Write Data to RAM Sel/1

== system CMOS_Kernel_Memory_Sync/Memory Handler/Memory Manager/Scanline Memory Subsystem ==
  Read Address : Inport
  Read Enable : Inport  Port=2
  Write Address : Inport  Port=3
  Write Data to RAM Sel : Inport  Port=4
  Data To Write : Inport  Port=5
  Write Enable : Inport  Port=6
  Convert to BOOL : hdlBasic/Convert  gui_display_data_type=Boolean  arith_type=Boolean  n_bits=16  bin_pt=14  float_type=Single  exp_bits=8  fraction_bits=24  quantization=Truncate  overflow=Wrap  en=off  latency=1  pipeline=off  XmcBlockStatus=1  maskContainerNames=group2  block_type=convert  block_config=sysgen:Convert_config  block_width=595  block_height=885
  Dual Port RAM {0..4} (5 alike) : hdlBasic/Dual Port RAM  depth=ScanlineRamDepth  initVector=sin(pi*(0:15)/16)  distributed_mem=Ultra RAM  init_a=0  init_b=0  rst_a=off  rst_b=off  en_a=on  en_b=on  latency=1  write_mode_A=Read After Write  write_mode_B=Read After Write  explicit_period=[]  period=[]  simulation_type=fast_sim  XmcBlockStatus=1  maskContainerNames=tabcontainer1  block_type=dpram  block_config=sysgen:Dpram_config  optimize=Area
      settings: infoedit=[]
  RAM Selector 0 : Subsystem
      settings: RTWMemSecFuncInitTerm=Inherit fRAM model  RTWMemSecFuncExecute=Inherit fRAM model  RTWMemSecDataConstants=Inherit fRAM model  RTWMemSecDataInternal=Inherit fRAM model  RTWMemSecDataParameters=Inherit fRAM model
  RAM Selector 1 : Subsystem
      settings: RTWMemSecFuncInitTerm=Inherit fRAM model  RTWMemSecFuncExecute=Inherit fRAM model  RTWMemSecDataConstants=Inherit fRAM model  RTWMemSecDataInternal=Inherit fRAM model  RTWMemSecDataParameters=Inherit fRAM model
  RAM Selector 2 : Subsystem
      settings: RTWMemSecFuncInitTerm=Inherit fRAM model  RTWMemSecFuncExecute=Inherit fRAM model  RTWMemSecDataConstants=Inherit fRAM model  RTWMemSecDataInternal=Inherit fRAM model  RTWMemSecDataParameters=Inherit fRAM model
  Read Constant : hdlBasic/Constant  const=0  gui_display_data_type=Boolean  arith_type=Boolean  n_bits=16  bin_pt=14  preci_type=Single  exp_width=8  frac_width=24  explicit_period=off  period=1  XmcBlockStatus=1  maskContainerNames=tabcontainer1  block_type=constant  block_config=sysgen:Constant_config
  Write Constant : hdlBasic/Constant  const=1.0  gui_display_data_type=Boolean  arith_type=Boolean  n_bits=16  bin_pt=14  preci_type=Single  exp_width=8  frac_width=24  explicit_period=off  period=1  XmcBlockStatus=1  maskContainerNames=tabcontainer1  block_type=constant  block_config=sysgen:Constant_config
  RAM 0 Out : Outport
  RAM 1 Out : Outport  Port=2
  RAM 2 Out : Outport  Port=3
  RAM 3 Out : Outport  Port=4
  RAM 4 Out : Outport  Port=5
  Valid : Outport  Port=6
  wires:
  RAM Selector 2/1(Out RAM 0) -> Dual Port RAM 0/8
  Dual Port RAM 1/1 -> RAM 1 Out/1
  RAM Selector 0/5(Out RAM 4) -> Dual Port RAM 4/4
  Write Constant/1 -> Dual Port RAM 4/6, Dual Port RAM 3/6, Dual Port RAM 2/6, Dual Port RAM 1/6, Dual Port RAM 0/6
  Read Constant/1 -> Dual Port RAM 4/3, Dual Port RAM 3/3, Dual Port RAM 2/3, Dual Port RAM 1/3, Dual Port RAM 0/3
  RAM Selector 1/4(Out RAM 3) -> Dual Port RAM 3/2, Dual Port RAM 3/5
  RAM Selector 0/2(Out RAM 1) -> Dual Port RAM 1/4
  RAM Selector 2/5(Out RAM 4) -> Dual Port RAM 4/8
  RAM Selector 0/4(Out RAM 3) -> Dual Port RAM 3/4
  RAM Selector 1/1(Out RAM 0) -> Dual Port RAM 0/2, Dual Port RAM 0/5
  RAM Selector 1/2(Out RAM 1) -> Dual Port RAM 1/2, Dual Port RAM 1/5
  RAM Selector 1/5(Out RAM 4) -> Dual Port RAM 4/2, Dual Port RAM 4/5
  RAM Selector 1/3(Out RAM 2) -> Dual Port RAM 2/2, Dual Port RAM 2/5
  Dual Port RAM 4/1 -> RAM 4 Out/1
  RAM Selector 0/1(Out RAM 0) -> Dual Port RAM 0/4
  RAM Selector 0/3(Out RAM 2) -> Dual Port RAM 2/4
  RAM Selector 2/2(Out RAM 1) -> Dual Port RAM 1/8
  RAM Selector 2/4(Out RAM 3) -> Dual Port RAM 3/8
  RAM Selector 2/3(Out RAM 2) -> Dual Port RAM 2/8
  Dual Port RAM 3/1 -> RAM 3 Out/1
  Dual Port RAM 2/1 -> RAM 2 Out/1
  Dual Port RAM 0/1 -> RAM 0 Out/1
  Write Enable/1 -> RAM Selector 2/1(Data In)
  Data To Write/1 -> RAM Selector 1/1(Data In)
  Write Address/1 -> RAM Selector 0/1(Data In)
  Write Data to RAM Sel/1 -> RAM Selector 0/2(RAM Select), RAM Selector 2/2(RAM Select), RAM Selector 1/2(RAM Select)
  Read Address/1 -> Dual Port RAM 0/1, Dual Port RAM 4/1, Dual Port RAM 3/1, Dual Port RAM 2/1, Dual Port RAM 1/1
  Read Enable/1 -> Convert to BOOL/1, Dual Port RAM 4/7, Dual Port RAM 3/7, Dual Port RAM 2/7, Dual Port RAM 1/7, Dual Port RAM 0/7
  Convert to BOOL/1 -> Valid/1
